simulink model "RobustDeviationDetection"  (R2024a)
settings: Solver=FixedStepAuto  StartTime=0.0  StopTime=200  FixedStep=0.01  RelTol=1e-3  EnableMultiTasking=on
libraries: AVE_Library x1
settings Model: Creator=damerius  LastModifiedBy=Scythe
settings SolverCC: ConcurrentTasks=on  AlgebraicLoopSolver=TrustRegion  PositivePriorityOrder=on
settings DataIOCC: SaveOutput=off  SignalLogging=off  DSMLogging=off  SaveTime=off  ReturnWorkspaceOutputs=off
settings OptimizationCC: DefaultParameterBehavior=Inlined  ReuseModelBlockBuffer=off  ZeroExternalMemoryAtStartup=off  ZeroInternalMemoryAtStartup=off  SimCompilerOptimization=on
settings DebuggingCC: UnconnectedInputMsg=warning  UnconnectedOutputMsg=warning  UnconnectedLineMsg=warning
settings HardwareCC: ProdBitPerLong=64  ProdHWDeviceType=Intel->x86-64 (Linux 64)
settings ModelReferenceCC: EnableRefExpFcnMdlSchedulingChecks=on
settings SFSimCC: SimParseCustomCode=off  SimGenImportedTypeDefs=on  SimTargetLang=C++
settings RTWCC: GenCodeOnly=on  PackageGeneratedCodeAndArtifacts=on  PackageName=PackNGo  RTWVerbose=off  BuildConfiguration=Faster Runs  TargetLang=C++  GPUComputeCapability=3.5  DLArmComputeVersion=19.05
settings CodeAppCC: ForceParamTrailComments=on  MaxIdLength=95  MATLABSourceComments=on  UseSimReservedNames=on
settings GRTTargetCC: TargetLangStandard=C++11 (ISO)  GenerateFullHeader=off  MatFileLogging=off  CodeInterfacePackaging=C++ class

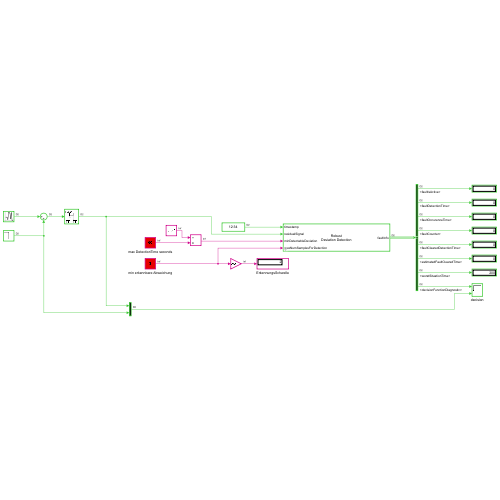
[thumbnail: Simulink's stored preview of the top-level diagram]
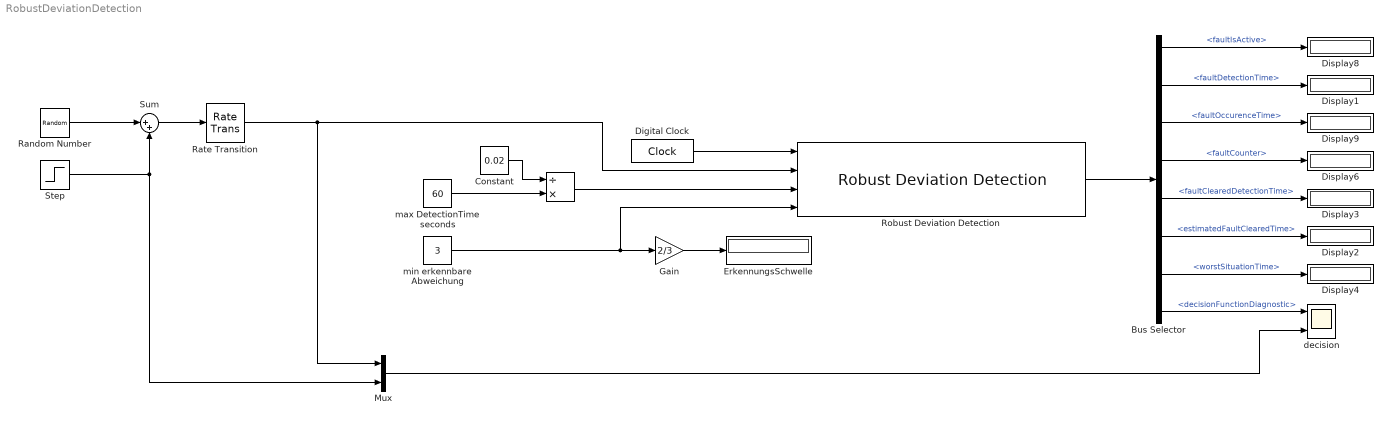
== system RobustDeviationDetection ==
  "  " : Product  Inputs=/*
  Bus Selector : BusSelector  OutputSignals=faultIsActive,faultDetectionTime,faultOccurenceTime,faultCounter,faultClearedDetectionTime,estimatedFaultClearedTime,worstSituationTime,decisionFunctionDiagnostic
  Constant : Constant  Value=0.02
  Digital Clock : DigitalClock  SampleTime=0.02
  Display{1..4,6,8..9} (7 alike) : Display
  ErkennungsSchwelle : Display
  Gain : Gain  Gain=2/3
  Mux : Mux  Inputs=2
  Random Number : RandomNumber  Variance=10*10  Seed=11  SampleTime=0.02
  Rate Transition : RateTransition  OutPortSampleTime=0.02
  Robust Deviation Detection : AVE_Library/Fault Detection and Isolation/Robust Deviation Detection
  Step : Step  Time=100  After=-3  SampleTime=0.02
  Sum : Sum  Inputs=|++
  decision : Scope  NumInputPorts=2
  max DetectionTime seconds : Constant  Value=60
  min erkennbare Abweichung : Constant  Value=3
  wires:
  Bus Selector/1 -> Display8/1  "<faultIsActive>"
  Robust Deviation Detection/1 -> Bus Selector/1
  Rate Transition/1 -> Robust Deviation Detection/2, Mux/1
  Bus Selector/8 -> decision/1  "<decisionFunctionDiagnostic>"
  Gain/1 -> ErkennungsSchwelle/1
  min erkennbare Abweichung/1 -> Robust Deviation Detection/4, Gain/1
  max DetectionTime seconds/1 -> "  "/2
  Random Number/1 -> Sum/1
  Bus Selector/5 -> Display3/1  "<faultClearedDetectionTime>"
  Bus Selector/6 -> Display2/1  "<estimatedFaultClearedTime>"
  Mux/1 -> decision/2
  Constant/1 -> "  "/1
  Step/1 -> Mux/2, Sum/2
  Bus Selector/2 -> Display1/1  "<faultDetectionTime>"
  Bus Selector/7 -> Display4/1  "<worstSituationTime>"
  "  "/1 -> Robust Deviation Detection/3
  Digital Clock/1 -> Robust Deviation Detection/1
  Bus Selector/3 -> Display9/1  "<faultOccurenceTime>"
  Bus Selector/4 -> Display6/1  "<faultCounter>"
  Sum/1 -> Rate Transition/1
